simulink model "First_order_simulink"  (R2020b)
settings: Solver=VariableStepAuto  StartTime=0.0  StopTime=100  RelTol=1e-3
settings Model: Creator=99003785  LastModifiedBy=99003785

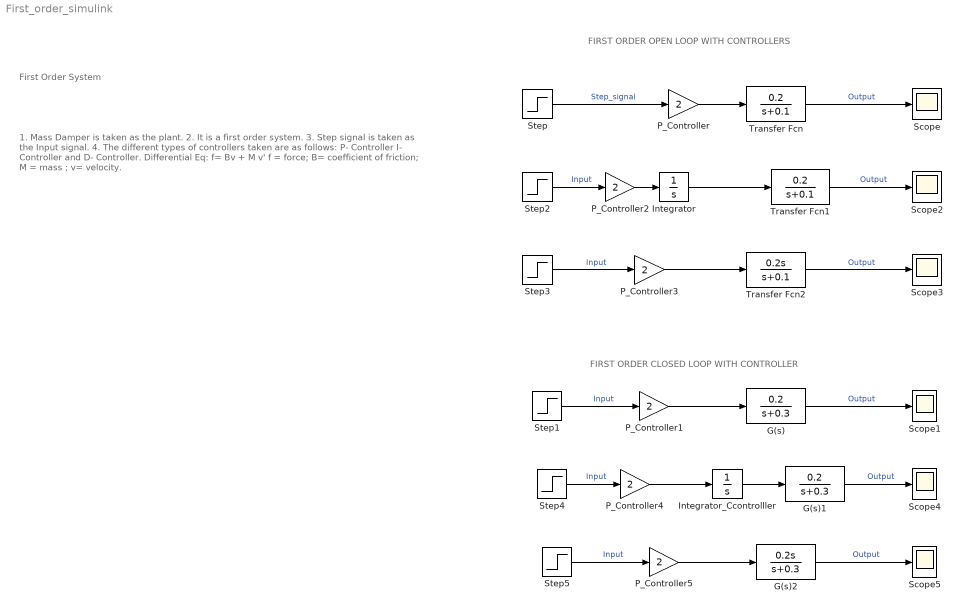
== system First_order_simulink ==
  note: 1. Mass Damper is taken as the plant.
      | 2. It is a first order system.
      | 3. Step signal is taken as the Input signal.
      | 4. The different types of controllers taken are as follows:
      | P- Controller I- Controller and D- Controller.
      |
      | Differential Eq: f= Bv + M v'
      | f = force; B= coefficient of friction; M = mass ; v= velocity.
  note: First Order System
  note: FIRST ORDER OPEN LOOP WITH CONTROLLERS
  note: FIRST ORDER CLOSED LOOP WITH CONTROLLER
  G(s) : TransferFcn  Numerator=[0.2]  Denominator=[1 0.3]
  G(s)1 : TransferFcn  Numerator=[0.2]  Denominator=[1 0.3]
  G(s)2 : TransferFcn  Numerator=[0.2,0]  Denominator=[1 0.3]
  Integrator : Integrator
  Integrator_Ccontrolller : Integrator
  P_Controller{,1..5} (6 alike) : Gain  Gain=2
  Scope{,1..5} (6 alike) : Scope
  Step{,1..5} (6 alike) : Step  SampleTime=0
  Transfer Fcn : TransferFcn  Numerator=[0.2]  Denominator=[1 0.1]
  Transfer Fcn1 : TransferFcn  Numerator=[0.2]  Denominator=[1 0.1]
  Transfer Fcn2 : TransferFcn  Numerator=[0.2,0]  Denominator=[1 0.1]
  wires:
  Transfer Fcn/1 -> Scope/1  "Output"
  P_Controller/1 -> Transfer Fcn/1
  Step/1 -> P_Controller/1  "Step_signal"
  G(s)/1 -> Scope1/1  "Output"
  Step1/1 -> P_Controller1/1  "Input"
  P_Controller1/1 -> G(s)/1
  Transfer Fcn1/1 -> Scope2/1  "Output"
  Integrator/1 -> Transfer Fcn1/1
  Step2/1 -> P_Controller2/1  "Input"
  P_Controller2/1 -> Integrator/1
  Transfer Fcn2/1 -> Scope3/1  "Output"
  Step3/1 -> P_Controller3/1  "Input"
  P_Controller3/1 -> Transfer Fcn2/1
  G(s)1/1 -> Scope4/1  "Output"
  Step4/1 -> P_Controller4/1  "Input"
  P_Controller4/1 -> Integrator_Ccontrolller/1
  Integrator_Ccontrolller/1 -> G(s)1/1
  G(s)2/1 -> Scope5/1  "Output"
  P_Controller5/1 -> G(s)2/1
  Step5/1 -> P_Controller5/1  "Input"
